simulink subsystem "Decentralized_LFT"  (R2022a)
settings: Solver=VariableStepAuto  StartTime=0.0  StopTime=10.0  RelTol=1e-3
values from neighbouring files (symbols this model uses):
  fil = 0.1    [Decen_control_prepare.m]    (also in control_demo_prepare.m = 0.0001; simulation_CPG.m = 0.0001)
  Kd1 = 1    [Decen_control_prepare.m]
  Kp1 = 5000    [Decen_control_prepare.m]
  kta = 0.001    [Decen_control_prepare.m]
  ktp = 1    [Decen_control_prepare.m]
  ktv = 0.1    [Decen_control_prepare.m]
  sat_ceiling = -sat_floor    (= 10)    [Decen_control_prepare.m]    (also in control_demo_prepare.m = 40; simulation_CPG.m = 40)
  sat_floor = -10    [Decen_control_prepare.m]    (also in control_demo_prepare.m = -40; simulation_CPG.m = -40)
  Tv = 1    [Decen_control_prepare.m]
settings Model: Creator=liltrump  LastModifiedBy=liltrump

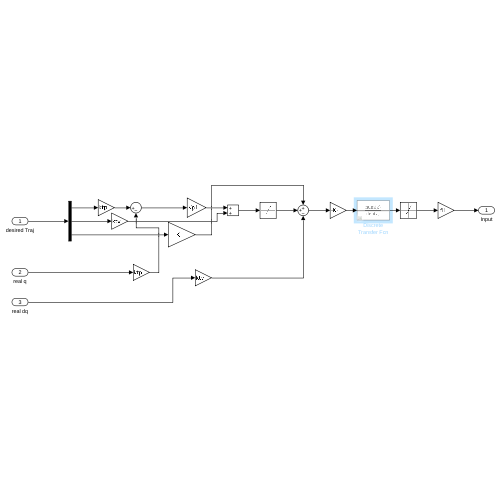
[thumbnail: Simulink's stored preview of the top-level diagram]
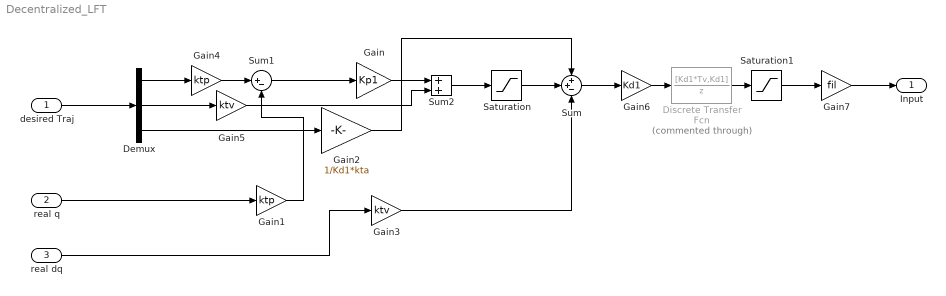
== system Decentralized_LFT ==
  desired Traj : Inport
  real q : Inport  Port=2
  real dq : Inport  Port=3
  Demux : Demux  Outputs=3
  Discrete Transfer Fcn : DiscreteTransferFcn  Commented=through  Numerator=[Kd1*Tv,Kd1]  Denominator=[1,0]
  Gain : Gain  Gain=Kp1
  Gain1 : Gain  Gain=ktp
  Gain2 : Gain  Gain=1/Kd1*kta
  Gain3 : Gain  Gain=ktv
  Gain4 : Gain  Gain=ktp
  Gain5 : Gain  Gain=ktv
  Gain6 : Gain  Gain=Kd1
  Gain7 : Gain  Gain=fil
  Saturation : Saturate  UpperLimit=sat_ceiling  LowerLimit=sat_floor
  Saturation1 : Saturate  UpperLimit=sat_ceiling*2  LowerLimit=sat_floor*2
  Sum : Sum  Inputs=++-
  Sum1 : Sum  Inputs=|+-
  Sum2 : Sum
  Input : Outport
  wires:
  desired Traj/1 -> Demux/1
  Sum1/1 -> Gain/1
  Gain/1 -> Sum2/1
  Gain2/1 -> Sum/1
  Sum2/1 -> Saturation/1
  Saturation/1 -> Sum/2
  Sum/1 -> Gain6/1
  Discrete Transfer Fcn/1 -> Saturation1/1
  Gain1/1 -> Sum1/2
  Gain3/1 -> Sum/3
  Gain4/1 -> Sum1/1
  Gain5/1 -> Sum2/2
  Demux/1 -> Gain4/1
  Demux/2 -> Gain5/1
  Demux/3 -> Gain2/1
  real q/1 -> Gain1/1
  real dq/1 -> Gain3/1
  Saturation1/1 -> Gain7/1
  Gain6/1 -> Discrete Transfer Fcn/1
  Gain7/1 -> Input/1
